simulink model "buck_boost_ccm_small"  (R2020a)
settings: Solver=VariableStepAuto  StartTime=0.0  StopTime=0.03  RelTol=1e-3
settings Model: Creator=ZLH  LastModifiedBy=robe

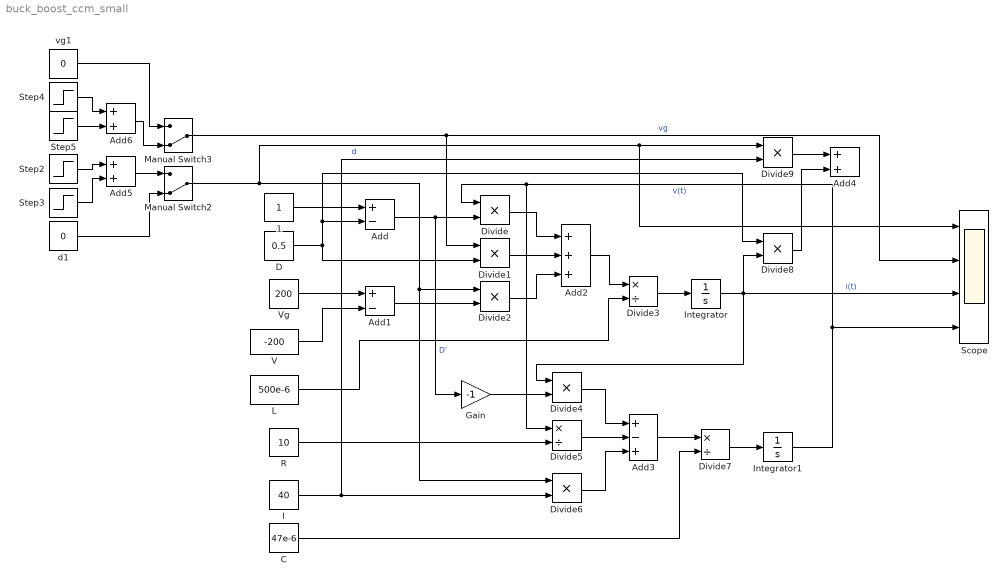
== system buck_boost_ccm_small ==
  1 : Constant
  Add : Sum  Inputs=+-
  Add1 : Sum  Inputs=+-
  Add2 : Sum  Inputs=+++
  Add3 : Sum  Inputs=+-+
  Add4 : Sum
  Add5 : Sum
  Add6 : Sum
  C : Constant  Value=47e-6
  D : Constant  Value=0.5
  Divide{,1..2,4,6,8..9} (7 alike) : Product  Inputs=**
  Divide3 : Product  Inputs=*/
  Divide5 : Product  Inputs=*/
  Divide7 : Product  Inputs=*/
  Gain : Gain  Gain=-1
  I : Constant  Value=40
  Integrator : Integrator
  Integrator1 : Integrator
  L : Constant  Value=500e-6
  Manual Switch2 : ManualSwitch  CurrentSetting=0
  Manual Switch3 : ManualSwitch  CurrentSetting=0
  R : Constant  Value=10
  Scope : Scope  NumInputPorts=4
  Step2 : Step  Time=0.01  After=0.02  SampleTime=0
  Step3 : Step  Time=0.02  After=-0.02  SampleTime=0
  Step4 : Step  Time=0.02  After=60  SampleTime=0
  Step5 : Step  Time=0.01  After=-60  SampleTime=0
  V : Constant  Value=-200
  Vg : Constant  Value=200
  d1 : Constant  Value=0
  vg1 : Constant  Value=0
  wires:
  Divide5/1 -> Add3/2
  D/1 -> Divide8/1, Add/2, Divide1/2
  Divide4/1 -> Add3/1
  Divide9/1 -> Add4/1
  Divide3/1 -> Integrator/1
  R/1 -> Divide5/2
  Gain/1 -> Divide4/2
  Integrator1/1 -> Scope/4, Divide/1, Divide5/1  "v(t)"
  L/1 -> Divide3/2
  Add/1 -> Gain/1, Divide/2  "D'"
  Manual Switch3/1 -> Scope/2, Divide1/1  "vg"
  Divide8/1 -> Add4/2
  I/1 -> Divide9/2, Divide6/2
  V/1 -> Add1/2
  Integrator/1 -> Scope/3, Divide8/2, Divide4/1  "i(t)"
  Divide/1 -> Add2/1
  C/1 -> Divide7/2
  Divide1/1 -> Add2/2
  Divide6/1 -> Add3/3
  Add3/1 -> Divide7/1
  Add1/1 -> Divide2/2
  Divide2/1 -> Add2/3
  Manual Switch2/1 -> Scope/1, Divide9/1, Divide6/1, Divide2/1  "d"
  Add2/1 -> Divide3/1
  1/1 -> Add/1
  Divide7/1 -> Integrator1/1
  Vg/1 -> Add1/1
  Step3/1 -> Add5/2
  Step4/1 -> Add6/1
  Add6/1 -> Manual Switch3/2
  Step5/1 -> Add6/2
  Step2/1 -> Add5/1
  d1/1 -> Manual Switch2/2
  Add5/1 -> Manual Switch2/1
  vg1/1 -> Manual Switch3/1
